simulink model "day1"  (R2024a)
settings: Solver=VariableStepAuto  StartTime=0.0  StopTime=10.0  RelTol=1e-3
settings Model: Creator=yasha  LastModifiedBy=tusha

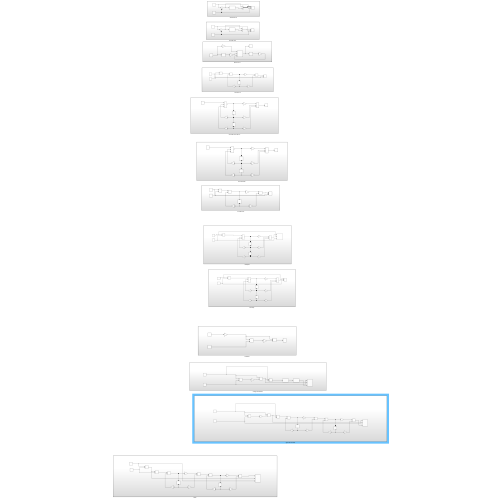
[thumbnail: Simulink's stored preview of the top-level diagram]
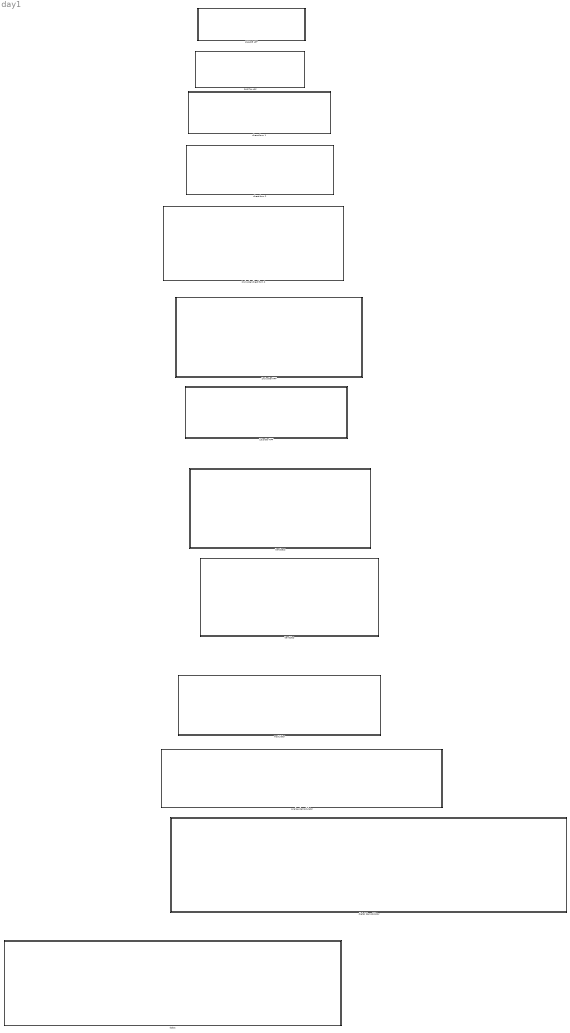
== system day1 ==
  1st order HPF : Subsystem
  2nd order HPF : Subsystem
  2nd order direct form 2 : Subsystem
  ANALOG LPF : Subsystem
  DIGITAL LPF : Subsystem
  analog demodulator : Subsystem
  "bandpass " : Subsystem
  bandstop : Subsystem
  digital demodulator : Subsystem
  direcrt form 1 : Subsystem
  direct form 2 : Subsystem
  dsbsc : Subsystem
  modulator : Subsystem

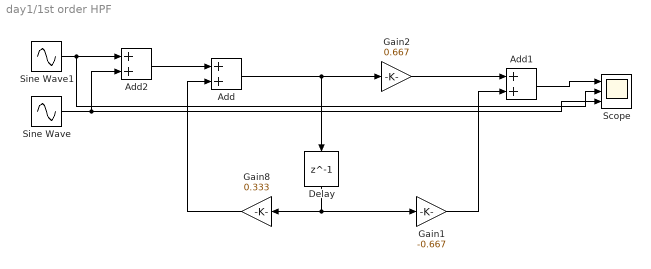
== system day1/1st order HPF ==
  Add : Sum
  Add1 : Sum
  Add2 : Sum
  Delay : Delay  DelayLength=1  InitialCondition=0
  Gain1 : Gain  Gain=-0.667
  Gain2 : Gain  Gain=0.667
  Gain8 : Gain  Gain=0.333
  Scope : Scope  NumInputPorts=3
  Sine Wave : Sin  Frequency=50  SampleTime=0
  Sine Wave1 : Sin  Frequency=5  SampleTime=0
  wires:
  Add/1 -> Delay/1, Gain2/1
  Gain2/1 -> Add1/1
  Add1/1 -> Scope/1
  Delay/1 -> Gain1/1, Gain8/1
  Gain8/1 -> Add/2
  Gain1/1 -> Add1/2
  Add2/1 -> Add/1
  Sine Wave1/1 -> Scope/2, Add2/1
  Sine Wave/1 -> Scope/3, Add2/2

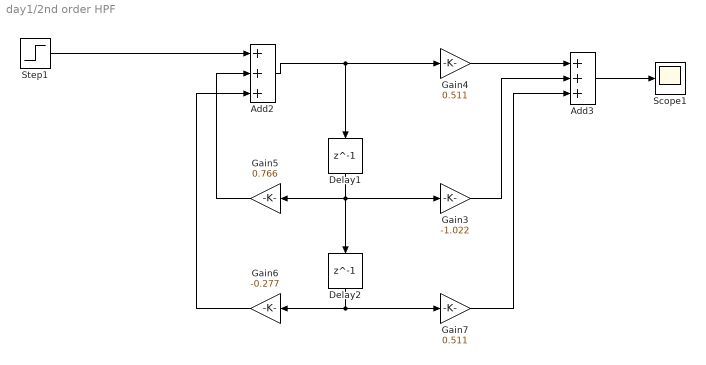
== system day1/2nd order HPF ==
  Add2 : Sum  Inputs=+++
  Add3 : Sum  Inputs=+++
  Delay1 : Delay  DelayLength=1  InitialCondition=0
  Delay2 : Delay  DelayLength=1  InitialCondition=0
  Gain3 : Gain  Gain=-1.022
  Gain4 : Gain  Gain=0.511
  Gain5 : Gain  Gain=0.766
  Gain6 : Gain  Gain=-0.277
  Gain7 : Gain  Gain=0.511
  Scope1 : Scope
  Step1 : Step  SampleTime=0
  wires:
  Step1/1 -> Add2/1
  Gain4/1 -> Add3/1
  Gain3/1 -> Add3/2
  Gain6/1 -> Add2/3
  Delay1/1 -> Delay2/1, Gain3/1, Gain5/1
  Add2/1 -> Delay1/1, Gain4/1
  Gain7/1 -> Add3/3
  Add3/1 -> Scope1/1
  Delay2/1 -> Gain6/1, Gain7/1
  Gain5/1 -> Add2/2

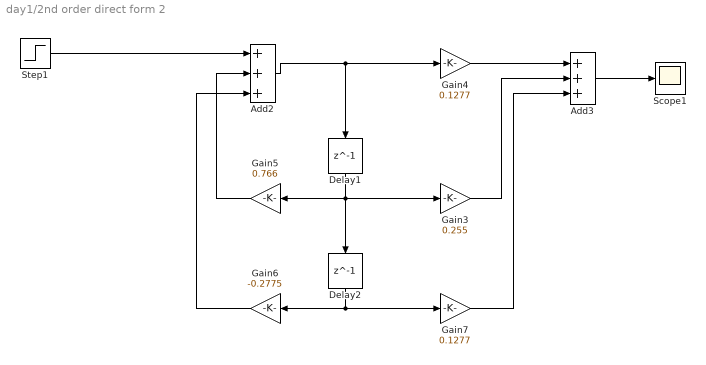
== system day1/2nd order direct form 2 ==
  Add2 : Sum  Inputs=+++
  Add3 : Sum  Inputs=+++
  Delay1 : Delay  DelayLength=1  InitialCondition=0
  Delay2 : Delay  DelayLength=1  InitialCondition=0
  Gain3 : Gain  Gain=0.255
  Gain4 : Gain  Gain=0.1277
  Gain5 : Gain  Gain=0.766
  Gain6 : Gain  Gain=-0.2775
  Gain7 : Gain  Gain=0.1277
  Scope1 : Scope
  Step1 : Step  SampleTime=0
  wires:
  Delay1/1 -> Delay2/1, Gain3/1, Gain5/1
  Add2/1 -> Delay1/1, Gain4/1
  Gain6/1 -> Add2/3
  Delay2/1 -> Gain6/1, Gain7/1
  Gain7/1 -> Add3/3
  Gain5/1 -> Add2/2
  Step1/1 -> Add2/1
  Add3/1 -> Scope1/1
  Gain3/1 -> Add3/2
  Gain4/1 -> Add3/1

== system day1/ANALOG LPF ==
  Bus Creator : BusCreator  Inputs=2
  Scope : Scope  NumInputPorts=3
  Sine Wave : Sin  SampleTime=0
  Sine Wave1 : Sin  Frequency=10  SampleTime=0
  Sum : Sum  Inputs=|++
  Transfer Fcn : TransferFcn  Denominator=[1 1]
  wires:
  Bus Creator/1 -> Scope/1
  Sine Wave/1 -> Scope/3, Sum/1
  Transfer Fcn/1 -> Bus Creator/2
  Sine Wave1/1 -> Scope/2, Sum/2
  Sum/1 -> Bus Creator/1, Transfer Fcn/1

== system day1/DIGITAL LPF ==
  Bus Creator1 : BusCreator  Inputs=2
  Discrete Transfer Fcn : DiscreteTransferFcn  Numerator=[0.0476 0.0476]  Denominator=[1 -0.9078]
  Scope1 : Scope  NumInputPorts=3
  Sine Wave2 : Sin  SampleTime=0
  Sine Wave3 : Sin  Frequency=10  SampleTime=0
  Sum1 : Sum  Inputs=|++
  wires:
  Sum1/1 -> Discrete Transfer Fcn/1, Bus Creator1/1
  Sine Wave3/1 -> Scope1/2, Sum1/2
  Sine Wave2/1 -> Scope1/3, Sum1/1
  Discrete Transfer Fcn/1 -> Bus Creator1/2
  Bus Creator1/1 -> Scope1/1

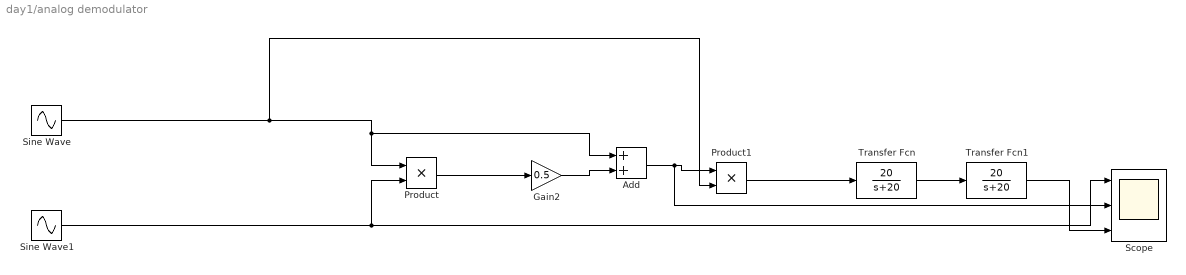
== system day1/analog demodulator ==
  Add : Sum
  Gain2 : Gain  Gain=0.5
  Product : Product
  Product1 : Product
  Scope : Scope  NumInputPorts=3
  Sine Wave : Sin  Amplitude=5  Frequency=100  SampleTime=0
  Sine Wave1 : Sin  SampleTime=0
  Transfer Fcn : TransferFcn  Numerator=[20]  Denominator=[1 20]
  Transfer Fcn1 : TransferFcn  Numerator=[20]  Denominator=[1 20]
  wires:
  Gain2/1 -> Add/2
  Sine Wave/1 -> Product1/2, Add/1, Product/1
  Transfer Fcn/1 -> Transfer Fcn1/1
  Sine Wave1/1 -> Scope/1, Product/2
  Product/1 -> Gain2/1
  Add/1 -> Scope/2, Product1/1
  Product1/1 -> Transfer Fcn/1
  Transfer Fcn1/1 -> Scope/3

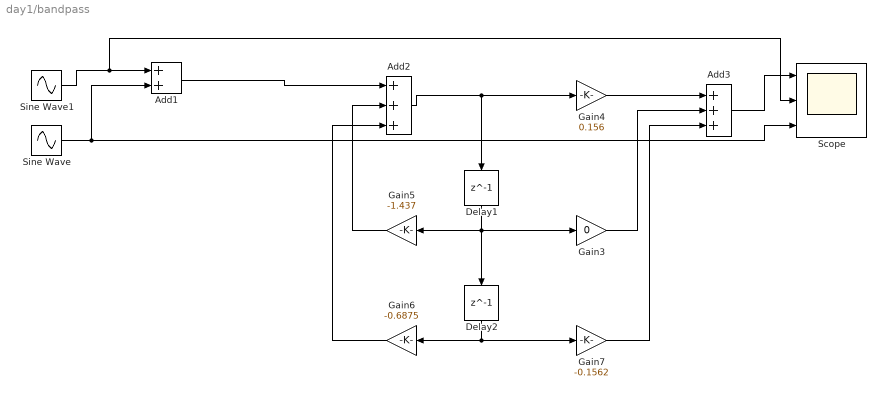
== system day1/bandpass  ==
  Add1 : Sum
  Add2 : Sum  Inputs=+++
  Add3 : Sum  Inputs=+++
  Delay1 : Delay  DelayLength=1  InitialCondition=0
  Delay2 : Delay  DelayLength=1  InitialCondition=0
  Gain3 : Gain  Gain=0
  Gain4 : Gain  Gain=0.156
  Gain5 : Gain  Gain=-1.437
  Gain6 : Gain  Gain=-0.6875
  Gain7 : Gain  Gain=-0.1562
  Scope : Scope  NumInputPorts=3
  Sine Wave : Sin  Frequency=50  SampleTime=0
  Sine Wave1 : Sin  Frequency=5  SampleTime=0
  wires:
  Add3/1 -> Scope/1
  Delay2/1 -> Gain6/1, Gain7/1
  Add2/1 -> Delay1/1, Gain4/1
  Gain7/1 -> Add3/3
  Gain6/1 -> Add2/3
  Add1/1 -> Add2/1
  Delay1/1 -> Delay2/1, Gain3/1, Gain5/1
  Gain5/1 -> Add2/2
  Gain4/1 -> Add3/1
  Gain3/1 -> Add3/2
  Sine Wave/1 -> Add1/2, Scope/3
  Sine Wave1/1 -> Scope/2, Add1/1

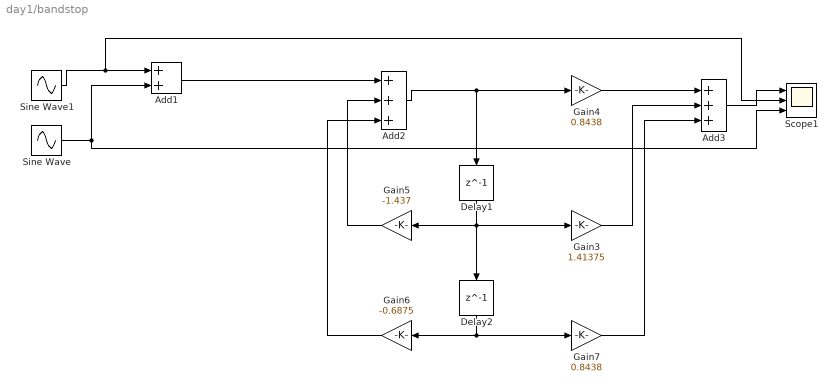
== system day1/bandstop ==
  Add1 : Sum
  Add2 : Sum  Inputs=+++
  Add3 : Sum  Inputs=+++
  Delay1 : Delay  DelayLength=1  InitialCondition=0
  Delay2 : Delay  DelayLength=1  InitialCondition=0
  Gain3 : Gain  Gain=1.41375
  Gain4 : Gain  Gain=0.8438
  Gain5 : Gain  Gain=-1.437
  Gain6 : Gain  Gain=-0.6875
  Gain7 : Gain  Gain=0.8438
  Scope1 : Scope  NumInputPorts=3
  Sine Wave : Sin  Frequency=50  SampleTime=0
  Sine Wave1 : Sin  Frequency=5  SampleTime=0
  wires:
  Add1/1 -> Add2/1
  Gain3/1 -> Add3/2
  Add2/1 -> Delay1/1, Gain4/1
  Gain6/1 -> Add2/3
  Delay1/1 -> Delay2/1, Gain3/1, Gain5/1
  Delay2/1 -> Gain6/1, Gain7/1
  Add3/1 -> Scope1/1
  Gain4/1 -> Add3/1
  Gain7/1 -> Add3/3
  Gain5/1 -> Add2/2
  Sine Wave1/1 -> Scope1/2, Add1/1
  Sine Wave/1 -> Add1/2, Scope1/3

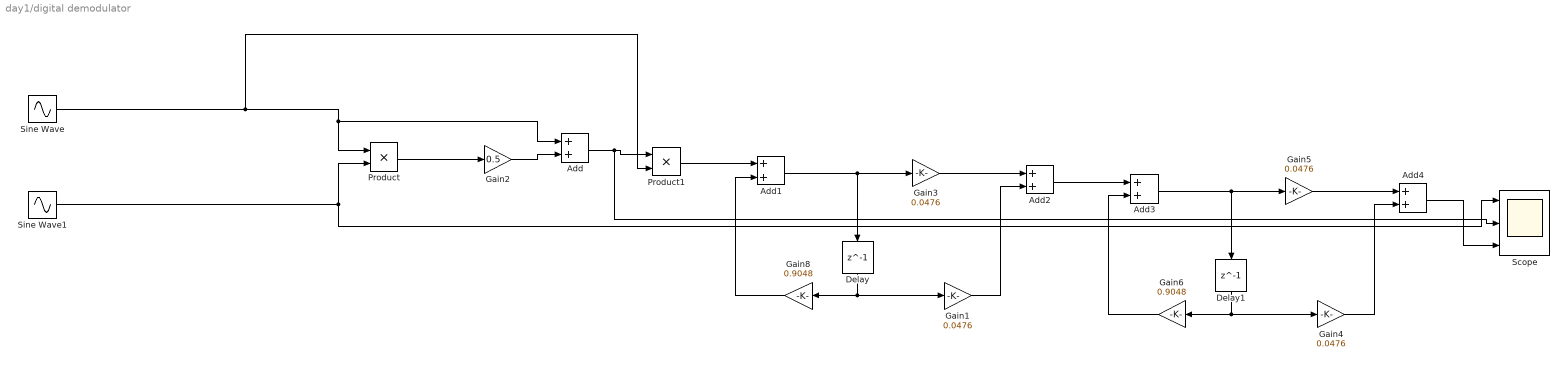
== system day1/digital demodulator ==
  Add{,1..4} (5 alike) : Sum
  Delay : Delay  DelayLength=1  InitialCondition=0
  Delay1 : Delay  DelayLength=1  InitialCondition=0
  Gain{1,3..5} (4 alike) : Gain  Gain=0.0476
  Gain2 : Gain  Gain=0.5
  Gain6 : Gain  Gain=0.9048
  Gain8 : Gain  Gain=0.9048
  Product : Product
  Product1 : Product
  Scope : Scope  NumInputPorts=3
  Sine Wave : Sin  Amplitude=5  Frequency=100  SampleTime=0
  Sine Wave1 : Sin  SampleTime=0
  wires:
  Add1/1 -> Delay/1, Gain3/1
  Delay/1 -> Gain1/1, Gain8/1
  Sine Wave/1 -> Product1/2, Add/1, Product/1
  Add/1 -> Scope/2, Product1/1
  Gain3/1 -> Add2/1
  Sine Wave1/1 -> Scope/1, Product/2
  Gain2/1 -> Add/2
  Gain4/1 -> Add4/2
  Product/1 -> Gain2/1
  Add2/1 -> Add3/1
  Gain1/1 -> Add2/2
  Add3/1 -> Delay1/1, Gain5/1
  Product1/1 -> Add1/1
  Gain8/1 -> Add1/2
  Delay1/1 -> Gain4/1, Gain6/1
  Gain5/1 -> Add4/1
  Gain6/1 -> Add3/2
  Add4/1 -> Scope/3

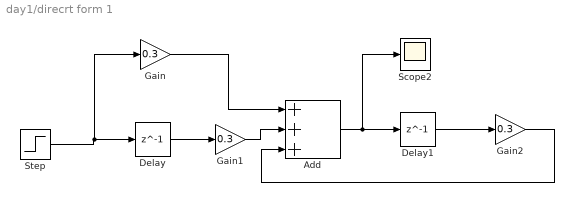
== system day1/direcrt form 1 ==
  Add : Sum  Inputs=+++
  Delay : Delay  DelayLength=1  InitialCondition=0
  Delay1 : Delay  DelayLength=1  InitialCondition=0
  Gain : Gain  Gain=0.3
  Gain1 : Gain  Gain=0.3
  Gain2 : Gain  Gain=0.3
  Scope2 : Scope
  Step : Step  SampleTime=0
  wires:
  Delay1/1 -> Gain2/1
  Delay/1 -> Gain1/1
  Step/1 -> Gain/1, Delay/1
  Gain/1 -> Add/1
  Gain1/1 -> Add/2
  Gain2/1 -> Add/3
  Add/1 -> Scope2/1, Delay1/1

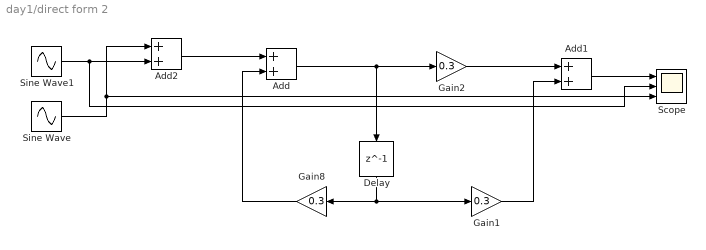
== system day1/direct form 2 ==
  Add : Sum
  Add1 : Sum
  Add2 : Sum
  Delay : Delay  DelayLength=1  InitialCondition=0
  Gain1 : Gain  Gain=0.3
  Gain2 : Gain  Gain=0.3
  Gain8 : Gain  Gain=0.3
  Scope : Scope  NumInputPorts=3
  Sine Wave : Sin  Frequency=50  SampleTime=0
  Sine Wave1 : Sin  Frequency=5  SampleTime=0
  wires:
  Gain1/1 -> Add1/2
  Delay/1 -> Gain1/1, Gain8/1
  Add1/1 -> Scope/1
  Gain8/1 -> Add/2
  Add/1 -> Delay/1, Gain2/1
  Gain2/1 -> Add1/1
  Add2/1 -> Add/1
  Sine Wave1/1 -> Scope/2, Add2/2
  Sine Wave/1 -> Scope/3, Add2/1

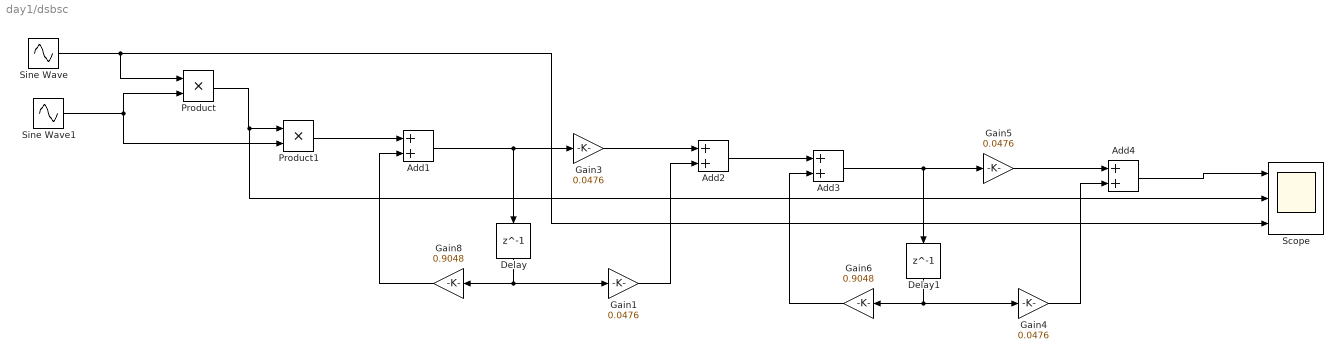
== system day1/dsbsc ==
  Add{1..4} (4 alike) : Sum
  Delay : Delay  DelayLength=1  InitialCondition=0
  Delay1 : Delay  DelayLength=1  InitialCondition=0
  Gain{1,3..5} (4 alike) : Gain  Gain=0.0476
  Gain6 : Gain  Gain=0.9048
  Gain8 : Gain  Gain=0.9048
  Product : Product
  Product1 : Product
  Scope : Scope  NumInputPorts=3
  Sine Wave : Sin  SampleTime=0
  Sine Wave1 : Sin  Frequency=100  SampleTime=0
  wires:
  Sine Wave/1 -> Scope/3, Product/1
  Gain4/1 -> Add4/2
  Delay1/1 -> Gain4/1, Gain6/1
  Add3/1 -> Delay1/1, Gain5/1
  Add4/1 -> Scope/1
  Gain6/1 -> Add3/2
  Product/1 -> Scope/2, Product1/1
  Gain5/1 -> Add4/1
  Gain1/1 -> Add2/2
  Gain3/1 -> Add2/1
  Gain8/1 -> Add1/2
  Add1/1 -> Delay/1, Gain3/1
  Delay/1 -> Gain1/1, Gain8/1
  Add2/1 -> Add3/1
  Sine Wave1/1 -> Product/2, Product1/2
  Product1/1 -> Add1/1

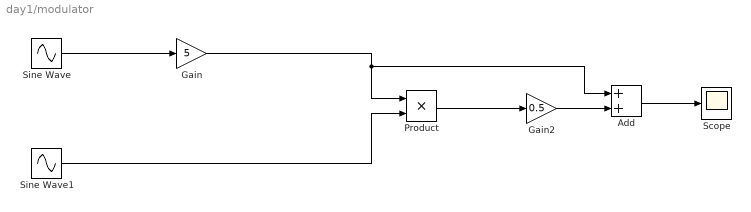
== system day1/modulator ==
  Add : Sum
  Gain : Gain  Gain=5
  Gain2 : Gain  Gain=0.5
  Product : Product
  Scope : Scope
  Sine Wave : Sin  Frequency=100  SampleTime=0
  Sine Wave1 : Sin  SampleTime=0
  wires:
  Gain/1 -> Add/1, Product/1
  Product/1 -> Gain2/1
  Add/1 -> Scope/1
  Gain2/1 -> Add/2
  Sine Wave1/1 -> Product/2
  Sine Wave/1 -> Gain/1
